simulink model "scheme1"  (R2024a)
settings: Solver=VariableStepAuto  StartTime=0.0  StopTime=20  RelTol=1e-9
values from neighbouring files (symbols this model uses):
  J = 0.0019    [main.m]
  ke = 0.3074    [main.m]
  km = 0.3074    [main.m]
  R = 4.6730    (= 4.673)    [main.m]
undefined symbols (not defined in the file or in its folder): func
settings Model: Creator=alexivanov  LastModifiedBy=alexivanov

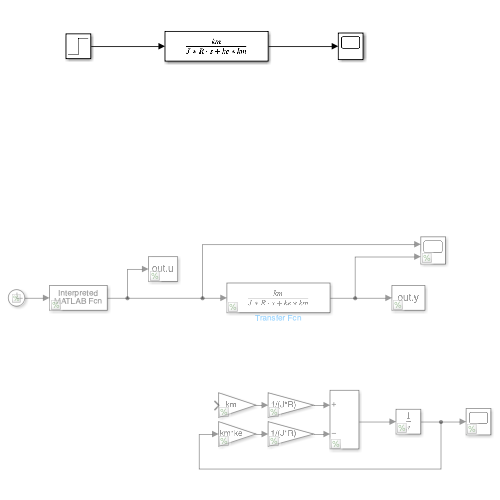
[thumbnail: Simulink's stored preview of the top-level diagram]
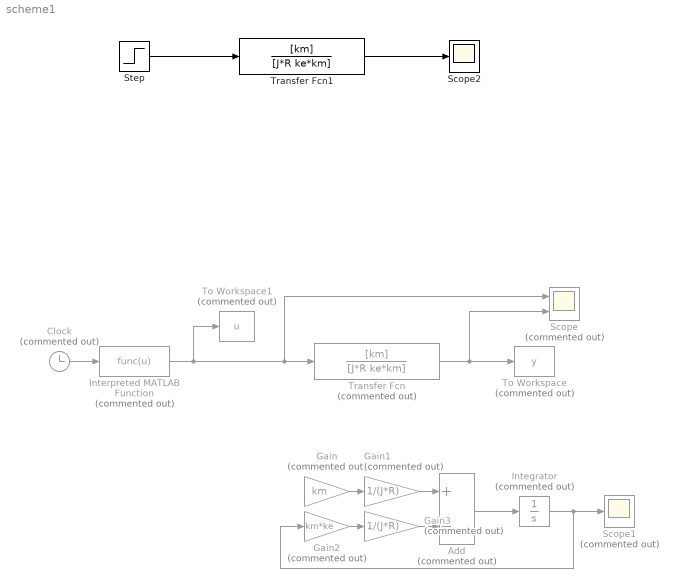
== system scheme1 ==
  Add : Sum  Commented=on  Inputs=+-
  Clock : Clock  Commented=on
  Gain : Gain  Commented=on  Gain=km
  Gain1 : Gain  Commented=on  Gain=1/(J*R)
  Gain2 : Gain  Commented=on  Gain=km*ke
  Gain3 : Gain  Commented=on  Gain=1/(J*R)
  Integrator : Integrator  Commented=on
  Interpreted MATLAB Function : MATLABFcn  Commented=on  MATLABFcn=func(u)
  Scope : Scope  Commented=on  NumInputPorts=2
  Scope1 : Scope  Commented=on
  Scope2 : Scope
  Step : Step  Time=0  SampleTime=0
  To Workspace : ToWorkspace  Commented=on  VariableName=y  SaveFormat=Timeseries  SampleTime=-1
  To Workspace1 : ToWorkspace  Commented=on  VariableName=u  SaveFormat=Timeseries  SampleTime=-1
  Transfer Fcn : TransferFcn  Commented=on  Numerator=[km]  Denominator=[J*R ke*km]
  Transfer Fcn1 : TransferFcn  Numerator=[km]  Denominator=[J*R ke*km]
  wires:
  Transfer Fcn/1 -> Scope/2, To Workspace/1
  Gain/1 -> Gain1/1
  Gain1/1 -> Add/1
  Gain2/1 -> Gain3/1
  Gain3/1 -> Add/2
  Add/1 -> Integrator/1
  Integrator/1 -> Gain2/1, Scope1/1
  Clock/1 -> Interpreted MATLAB Function/1
  Interpreted MATLAB Function/1 -> To Workspace1/1, Scope/1, Transfer Fcn/1
  Step/1 -> Transfer Fcn1/1
  Transfer Fcn1/1 -> Scope2/1
